simulink library "mag_vec_lib"  (R2016b)
settings: Solver=VariableStepAuto  StartTime=0.0  StopTime=10.0  RelTol=1e-3
undefined symbols (not defined in the file or in its folder): Earth, sim_params, WGS84
libraries: aerolibtransform2 x2, dspmathops x1, aerolibgravity2 x1, YMDHMS_2_dec_year x1
settings Model: Creator=Taylor  LastModifiedBy=evich

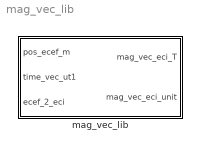
== system mag_vec_lib ==
  mag_vec_lib : Subsystem

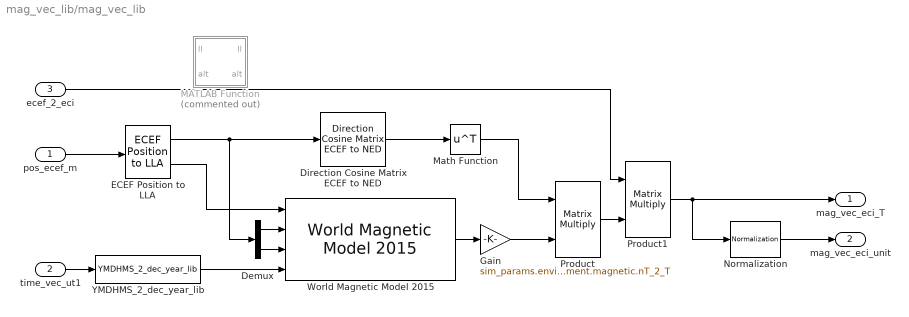
== system mag_vec_lib/mag_vec_lib ==
  pos_ecef_m : Inport
  time_vec_ut1 : Inport  Port=2
  ecef_2_eci : Inport  Port=3
  Demux : Demux  Outputs=2
  Direction Cosine Matrix ECEF to NED : aerolibtransform2/Direction Cosine Matrix ECEF to NED
  ECEF Position to LLA : aerolibtransform2/ECEF Position to LLA  units=Metric (MKS)  ptype=Earth (WGS84)  F=1/298.257223563  R=6378137
  Gain : Gain  Gain=sim_params.environment.magnetic.nT_2_T
  MATLAB Function : MATLAB Function  Commented=on  TreatAsAtomicUnit=on
  Math Function : Math  Operator=transpose  SaturateOnIntegerOverflow=on
  Normalization : dspmathops/Normalization  NormType=2-norm  Bias=1e-10  NormOver=Each column  Dimension=1  outputDataTypeStr=Inherit: Same as product output  outputLastDataTypeStr=Inherit: Same as product output  outputMin=[]  outputMax=[]  accumDataTypeStr=Inherit: Same as product output  accumLastDataTypeStr=Inherit: Same as product output  roundingMode=Floor  overflowMode=off
  Product : Product  Multiplication=Matrix(*)
  Product1 : Product  Multiplication=Matrix(*)
  World Magnetic Model 2015 : aerolibgravity2/World Magnetic Model 2015  units=Metric (MKS)  time_in=on  month=January  day=1  year=2015  action=None  h_out=off  dec_out=off  inc_out=off  ti_out=off
  YMDHMS_2_dec_year_lib : YMDHMS_2_dec_year/YMDHMS_2_dec_year_lib
  mag_vec_eci_T : Outport
  mag_vec_eci_unit : Outport  Port=2
  wires:
  ECEF Position to LLA/1 -> Demux/1, Direction Cosine Matrix ECEF to NED/1
  ECEF Position to LLA/2 -> World Magnetic Model 2015/1
  pos_ecef_m/1 -> ECEF Position to LLA/1
  World Magnetic Model 2015/1 -> Gain/1
  Gain/1 -> Product/2
  Direction Cosine Matrix ECEF to NED/1 -> Math Function/1
  Demux/1 -> World Magnetic Model 2015/2
  Demux/2 -> World Magnetic Model 2015/3
  Math Function/1 -> Product/1
  Product/1 -> Product1/2
  ecef_2_eci/1 -> Product1/1
  Product1/1 -> Normalization/1, mag_vec_eci_T/1
  Normalization/1 -> mag_vec_eci_unit/1
  YMDHMS_2_dec_year_lib/1 -> World Magnetic Model 2015/4
  time_vec_ut1/1 -> YMDHMS_2_dec_year_lib/1

== matlab function mag_vec_lib/MATLAB Function ==
  data: ll output; ll input; alt input; alt output
function [ll,alt] = fcn(ll,alt)
% If altitude is NaN, which should ONLY happen in first 1s when simulink is
% propagating signals and messes this one up.
%
% HuskySat-1, ADCS Subsystem
% T. Reynolds 12.18.17

if( isnan(alt) )
    alt = 5e5;
end

if( isnan(ll(1)) )
    ll(1) = 45;
end

if( isnan(ll(2)) )
   ll(2) = 90;
end
    
end
